simulink model "Simple_Pendulum"  (R2021a)
settings: Solver=VariableStepAuto  StartTime=0.0  StopTime=10.0  MaxStep=.001  RelTol=1e-3
settings Model: Creator=Admin  LastModifiedBy=Admin

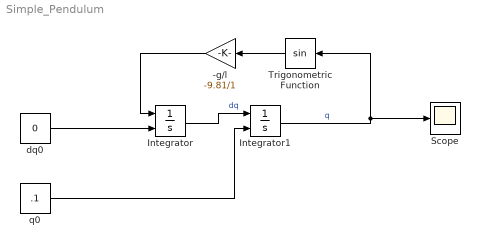
== system Simple_Pendulum ==
  -g/l : Gain  Gain=-9.81/1
  Integrator : Integrator  InitialConditionSource=external
  Integrator1 : Integrator  InitialConditionSource=external
  Scope : Scope
  Trigonometric Function : Trigonometry
  dq0 : Constant  Value=0
  q0 : Constant  Value=.1
  wires:
  Integrator/1 -> Integrator1/1  "dq"
  Integrator1/1 -> Scope/1, Trigonometric Function/1  "q"
  -g/l/1 -> Integrator/1
  Trigonometric Function/1 -> -g/l/1
  dq0/1 -> Integrator/2
  q0/1 -> Integrator1/2
